simulink model "Schemata"  (R2018a)
settings: Solver=VariableStepAuto  StartTime=0.0  StopTime=czas  RelTol=1e-3
values from neighbouring files (symbols this model uses):
  A = [(-cp*rop*fk-ks1-k0)/Cv1, k0/Cv1; (cp*rop*fk+k0)/Cv2, (-k0-cp*rop*fk-ks2)/Cv2]    [Skrypt.m]
  B = [cp*rop*fk/Cv1, ks1/Cv1; 0, ks2/Cv2]    [Skrypt.m]
  C = [1,0; 0,1]    [Skrypt.m]
  czas_skok = 50000    [Skrypt.m]
  D = [0,0; 0,0]    [Skrypt.m]
  dTkz0 = 0    [Skrypt.m]
  dTzew0 = 0    [Skrypt.m]
  Tkz0 = Tkzn * 1.0    (= 30)    [Skrypt.m]
  Tzew0 = Tzewn + 0    (= -20)    [Skrypt.m]
  x0 = -A^-1 * B*u0    [Skrypt.m]
settings Model: Creator=Mutungamiri  LastModifiedBy=Mutungamiri

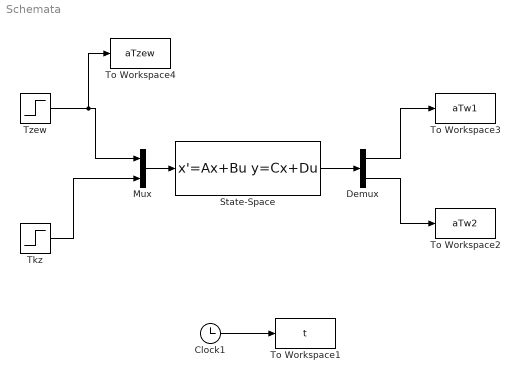
== system Schemata ==
  Clock1 : Clock
  Demux : Demux  Outputs=2
  Mux : Mux  Inputs=2
  State-Space : StateSpace  A=A  B=B  C=C  D=D  InitialCondition=x0
  Tkz : Step  Time=czas_skok  Before=Tkz0  After=Tkz0+dTkz0  SampleTime=0
  To Workspace1 : ToWorkspace  VariableName=t  SampleTime=-1
  To Workspace2 : ToWorkspace  VariableName=aTw2  SampleTime=-1
  To Workspace3 : ToWorkspace  VariableName=aTw1  SampleTime=-1
  To Workspace4 : ToWorkspace  VariableName=aTzew  SampleTime=-1
  Tzew : Step  Time=czas_skok  Before=Tzew0  After=Tzew0+dTzew0  SampleTime=0
  wires:
  Tzew/1 -> To Workspace4/1, Mux/1
  Tkz/1 -> Mux/2
  Demux/1 -> To Workspace3/1
  Demux/2 -> To Workspace2/1
  Mux/1 -> State-Space/1
  State-Space/1 -> Demux/1
  Clock1/1 -> To Workspace1/1
